simulink model "simProcObsStep"  (R2019a)
settings: Solver=FixedStepAuto  StartTime=0.0  StopTime=8  FixedStep=0.002  RelTol=1e-3
values from neighbouring files (symbols this model uses):
  A = [-4 -0.03; 0.75 -10]    [MDLsisotool.m]    (also in dadosSS.mat = [-31.7887619239  -14.7359524048; 16  0])
  B = [2; 0]    [MDLsisotool.m]    (also in dadosSS.mat = [16 0])
  C = [0 1]    [MDLsisotool.m]    (also in dadosSS.mat = [0 22.1495321335])
  D = 0    [MDLsisotool.m]    (also in dadosSS.mat)
  Ki = Kext(3)    [MDLsspace.m]    (also in dadosSS.mat = -0.0370352066606; ssGera.m)
  Kproc = [Kext(1), Kext(2)]    [MDLsspace.m]    (also in dadosSS.mat = [-0.861797620241 -0.503028275301]; ssGera.m)
  L = (acker(A', C', polosObs))'    [MDLsspace.m]    (also in dadosSS.mat = [-0.306409103952 0.415866033676]; ssGera.m)
settings Model: Creator=Cadu  LastModifiedBy=Cadu

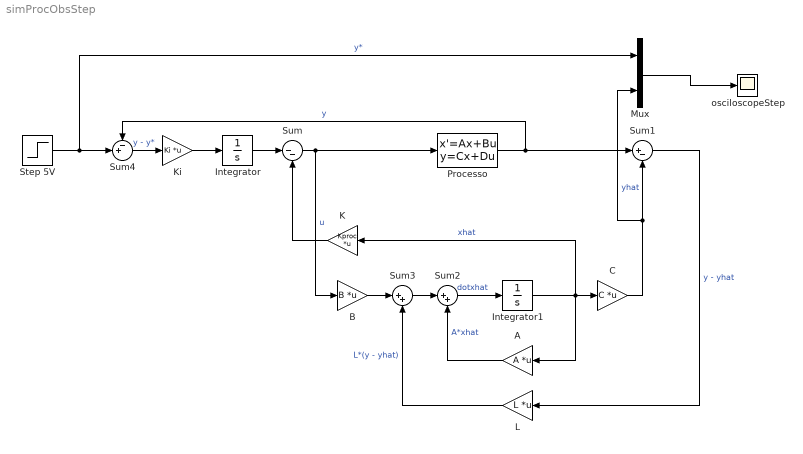
== system simProcObsStep ==
  " A" : Gain  Gain=A  Multiplication=Matrix(K*u)
  " K" : Gain  Gain=Kproc  Multiplication=Matrix(K*u)
  "B " : Gain  Gain=B  Multiplication=Matrix(K*u)
  C : Gain  Gain=C  Multiplication=Matrix(K*u)
  Integrator : Integrator
  Integrator1 : Integrator
  Ki : Gain  Gain=Ki  Multiplication=Matrix(K*u)
  "L " : Gain  Gain=L  Multiplication=Matrix(K*u)
  Mux : Mux  Inputs=2
  "Processo " : StateSpace  A=A  B=B  C=C  D=D  InitialCondition=0
  Step 5V : Step  Time=0.2  After=5  SampleTime=0
  Sum : Sum  Inputs=|--
  Sum1 : Sum  Inputs=|+-
  Sum2 : Sum  Inputs=|++
  Sum3 : Sum  Inputs=|++
  Sum4 : Sum  Inputs=-+|
  osciloscopeStep : Scope
  wires:
  Sum/1 -> "Processo "/1, "B "/1  "u"
  Integrator/1 -> Sum/1
  "Processo "/1 -> Sum1/1, Sum4/1  "y"
  Sum1/1 -> "L "/1  "y - yhat"
  Integrator1/1 -> " A"/1, C/1, " K"/1  "xhat"
  Sum2/1 -> Integrator1/1  "dotxhat"
  " K"/1 -> Sum/2
  Sum3/1 -> Sum2/1
  "B "/1 -> Sum3/1
  C/1 -> Mux/2, Sum1/2  "yhat"
  " A"/1 -> Sum2/2  "A*xhat"
  "L "/1 -> Sum3/2  "L*(y - yhat)"
  Ki/1 -> Integrator/1
  Mux/1 -> osciloscopeStep/1
  Step 5V/1 -> Sum4/2, Mux/1  "y*"
  Sum4/1 -> Ki/1  "y - y*"
